simulink model "Task_No6_R2023a"  (R2023a)
settings: Solver=ode5  StartTime=0.0  StopTime=3600*24*7  FixedStep=1  RelTol=1e-3
InitFcn:
  | PARAMETERS;
StartFcn:
  | PARAMETERS;
values from neighbouring files (symbols this model uses):
  Conv_C_to_K = 273.15    [PARAMETERS.m]
  P_AC_AIR_FLOW = 1    [PARAMETERS.m]
  P_CP_AIR = 1012    [PARAMETERS.m]
  P_DENSITY_AIR = 1.2041    [PARAMETERS.m]
  P_DENSITY_BRICK = 2/(10^-3)    (= 2000)    [PARAMETERS.m]
  P_DENSITY_PUR = 150    [PARAMETERS.m]
  P_EM_GLASS = 0.94    [PARAMETERS.m]
  P_EM_WALL = 0.94    [PARAMETERS.m]
  P_HANDLER_AIR_FLOW = 0.1    [PARAMETERS.m]
  P_HUMAN = 100    [PARAMETERS.m]
  P_INIT_CO2 = 420    [PARAMETERS.m]
  P_M_HUMAN_CO2 = 0.02*P_DENSITY_CO2/3600    (= 1.1e-05)    [PARAMETERS.m]
  P_M_HUMAN_VAPOR = 500*10^-3/(24*3600)    (= 5.78703703704e-06)    [PARAMETERS.m]
  P_M_WINDOW_SPEC = 20    [PARAMETERS.m]
  P_THICK_BRICK = 0.175    [PARAMETERS.m]
  P_THICK_PUR = P_THICK_WALL - P_THICK_BRICK    (= 0.125)    [PARAMETERS.m]
  RH_INIT_BDR = 40    [PARAMETERS.m]
  T_BREATH = 34    [PARAMETERS.m]
  T_COOLER = 12    [PARAMETERS.m]
  T_HEATER = 50    [PARAMETERS.m]
  T_INIT_BDR = 22    [PARAMETERS.m]
  T_INIT_OUT = 2.9    [PARAMETERS.m]
  U_WALL = 0.32    [PARAMETERS.m]
  U_WINDOW = 3.0    (= 3)    [PARAMETERS.m]
undefined symbols (not defined in the file or in its folder): P_AREA_BATH, P_AREA_BDR1, P_AREA_BDR2, P_AREA_EAST_WALL_BATH, P_AREA_EAST_WALL_BDR2, P_AREA_EAST_WALL_KIT, P_AREA_HALL, P_AREA_KIT, P_AREA_LVR, P_AREA_NORTH_WALL_BATH, P_AREA_NORTH_WALL_BDR1, P_AREA_NORTH_WALL_BDR2, P_AREA_OUTER_WALL_BATH, P_AREA_OUTER_WALL_BDR1, P_AREA_OUTER_WALL_BDR2, P_AREA_OUTER_WALL_HALL, P_AREA_OUTER_WALL_KIT, P_AREA_OUTER_WALL_LVR, P_AREA_SOUTH_WALL_KIT, P_AREA_SOUTH_WALL_LVR, P_AREA_WALL_BATH_KIT, P_AREA_WALL_BDR1_BDR2, P_AREA_WALL_BDR1_HALL, P_AREA_WALL_BDR2_BATH, P_AREA_WALL_BDR2_HALL, P_AREA_WALL_HALL_BATH, P_AREA_WALL_HALL_LVR, P_AREA_WALL_LVR_KIT, P_AREA_WIN_BATH, P_AREA_WIN_BDRS, P_AREA_WIN_KIT, P_AREA_WIN_LVR, P_M_AIR_BATH, P_M_AIR_BDR1, P_M_AIR_BDR2, P_M_AIR_HALL, P_M_AIR_KIT, P_M_AIR_LVR, TBL_SOL_EAST_01, TBL_SOL_EAST_02, TBL_SOL_EAST_03, TBL_SOL_EAST_04, TBL_SOL_EAST_05, TBL_SOL_EAST_06, TBL_SOL_EAST_07, TBL_SOL_EAST_08, TBL_SOL_EAST_09, TBL_SOL_EAST_10, TBL_SOL_EAST_11, TBL_SOL_EAST_12, TBL_SOL_NORTH_01, TBL_SOL_NORTH_02, TBL_SOL_NORTH_03, TBL_SOL_NORTH_04, TBL_SOL_NORTH_05, TBL_SOL_NORTH_06, TBL_SOL_NORTH_07, TBL_SOL_NORTH_08, TBL_SOL_NORTH_09, TBL_SOL_NORTH_10 ... (+7)
libraries: fl_lib x166, nesl_utility x88, slpidlib x3
(part 3 of 5)

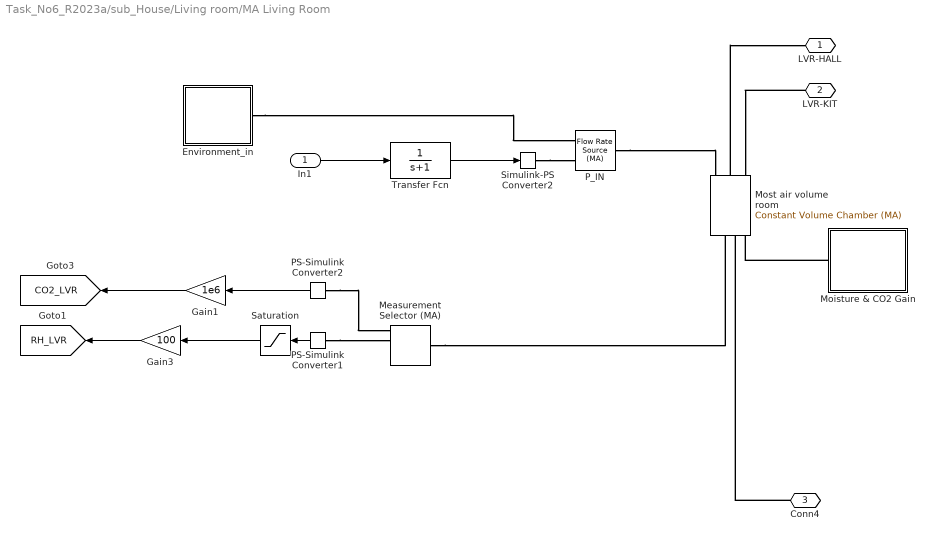
== system Task_No6_R2023a/sub_House/Living room/MA Living Room ==
  In1 : Inport
  Environment_in : Subsystem
  Gain1 : Gain  Gain=1e6
  Gain3 : Gain  Gain=100
  Measurement Selector (MA) : fl_lib/Moist Air/Sensors/Measurement Selector (MA)  moisture_spec=foundation.enum.moisture_spec.relative_humidity  trace_gas_spec=foundation.enum.trace_gas_spec.mass_fraction
  Moisture & CO2 Gain : Subsystem
  Most air volume room : fl_lib/Moist Air/Elements/Constant Volume Chamber (MA)  volume=P_M_AIR_LVR/P_DENSITY_AIR m^3  num_ports=foundation.enum.num_ports.three  area_A=P_AREA_DUCT m^2  area_B=P_AREA_DBL_DOOR m^2  area_C=P_AREA_DBL_DOOR m^2  area_D=0.01 m^2  RH_ws=1  time_constant=1 s  moisture_trace_gas_source=foundation.enum.moisture_trace_gas_source.controlled  moisture_source_spec=foundation.enum.moisture_source_spec.vapor  moisture_mass_flow=0 kg/s  moisture_temperature_spec=foundation.enum.temperature_spec.atmospheric  moisture_temperature=293.15 K  trace_gas_mass_flow=0 kg/s  trace_gas_temperature_spec=foundation.enum.temperature_spec.atmospheric  trace_gas_temperature=293.15 K  p_I_specify=on  p_I_priority=High  p_I=0.101325 MPa  p_I_nominal_specify=off  p_I_nominal_unit=MPa  p_I_nominal_value=1  T_I_specify=on  T_I_priority=High  T_I=T_INIT_BDR degC  T_I_nominal_specify=off  T_I_nominal_unit=K  T_I_nominal_value=1  RH_I_specify=on  RH_I_priority=High  RH_I=RH_INIT_BDR/100  RH_I_nominal_specify=off  RH_I_nominal_unit=1  RH_I_nominal_value=1  x_w_I_specify=off  x_w_I_priority=None  x_w_I=0  x_w_I_nominal_specify=off  x_w_I_nominal_unit=1  x_w_I_nominal_value=1  y_w_I_specify=off  y_w_I_priority=None  y_w_I=0  y_w_I_nominal_specify=off  y_w_I_nominal_unit=1  y_w_I_nominal_value=1  HR_I_specify=off  HR_I_priority=None  HR_I=0  HR_I_nominal_specify=off  HR_I_nominal_unit=1  HR_I_nominal_value=1  x_g_I_specify=on  x_g_I_priority=High  x_g_I=P_INIT_CO2/1e6  x_g_I_nominal_specify=off  x_g_I_nominal_unit=1  x_g_I_nominal_value=1  y_g_I_specify=off  y_g_I_priority=None  y_g_I=0  y_g_I_nominal_specify=off  y_g_I_nominal_unit=1  y_g_I_nominal_value=1
      settings: InternalSimscapePortConfiguration="{\"Bottom\":[],\"Left\":[{\"id\":\"A\",\"label\":\"A\",\"type\":\"foundation.moist_air.moist_air\"},{\"id\":\"B\",\"label\":\"B\",\"type\":\"foundation.moist_air.moist_air\"},{\"id\":\"C\",\"label\":\"C\",\"type\":\"foundation.moist_air.moist_air\"}],\"Right\":[{\"id\":\"W\",\"label\":\"W\",\"type\":\"output\"},{\"id\":\"F\",\"label\":\"F\",\"type\":\"output\"},{\"id\":\"H\",\"label\":\"H\",\"type\":\"foundation.thermal.thermal\"},{\"id\":\"S\",\"label\":\"S\",\"type\":\"foundation.moist_air.moist_air_source\"}],\"Top\":[]}"
  PS-Simulink Converter1 : nesl_utility/PS-Simulink Converter  PhysicalDomain=network_engine_domain  SubClassName=ps_output  LeftPortType=input  RightPortType=output  PseudoPeriodic=off  Frequencies=[]  VectorFormat=inherit  Unit=inherit  AffineConversion=off
  PS-Simulink Converter2 : nesl_utility/PS-Simulink Converter  PhysicalDomain=network_engine_domain  SubClassName=ps_output  LeftPortType=input  RightPortType=output  PseudoPeriodic=off  Frequencies=[]  VectorFormat=inherit  Unit=inherit  AffineConversion=off
  P_IN : fl_lib/Moist Air/Sources/Flow Rate Source (MA)  source_type=foundation.enum.constant_controlled.controlled  flow_type=foundation.enum.mass_volumetric_flow.mass  mass_flow=0 kg/s  volumetric_flow=0 m^3/s  volumetric_flow_conditions=foundation.enum.volumetric_flow_conditions.actual  p_std=0.101325 MPa  T_std=20 degC  RH_std=0.65  power_spec=foundation.enum.power_spec.isentropic  area_A=P_AREA_DUCT m^2  area_B=P_AREA_DUCT m^2
      settings: InternalSimscapePortConfiguration="{\"Bottom\":[],\"Left\":[{\"id\":\"A\",\"label\":\"A\",\"type\":\"foundation.moist_air.moist_air\"},{\"id\":\"M\",\"label\":\"M\",\"type\":\"input\"}],\"Right\":[{\"id\":\"B\",\"label\":\"B\",\"type\":\"foundation.moist_air.moist_air\"}],\"Top\":[]}"
  Saturation : Saturate  UpperLimit=1  LowerLimit=0
  Simulink-PS Converter2 : nesl_utility/Simulink-PS Converter  PhysicalDomain=network_engine_domain  SubClassName=ps_input  LeftPortType=input  RightPortType=output  PseudoPeriodic=off  Frequencies=[]  NoiseDistribution=none  NoiseParameters=[]  Unit=1  AffineConversion=off  FilteringAndDerivatives=provide  SimscapeFilterOrder=1  InputFilterTimeConstant=0.001  UdotUserProvided=0
  Transfer Fcn : TransferFcn  Denominator=[1 1]
  LVR-HALL : PMIOPort  Side=Left
  LVR-KIT : PMIOPort  Port=2  Side=Left
  Conn4 : PMIOPort  Port=3  Side=Right
  tag scope: CO2_LVR=global, RH_LVR=global
  wires:
  PS-Simulink Converter1/1 -> Saturation/1
  PS-Simulink Converter2/1 -> Gain1/1
  Saturation/1 -> Gain3/1
  Gain3/1 -> [RH_LVR]
  Gain1/1 -> [CO2_LVR]
  In1/1 -> Transfer Fcn/1
  Transfer Fcn/1 -> Simulink-PS Converter2/1
  connections:
  PS-Simulink Converter1/LConn1 -- Measurement Selector (MA)/RConn3
  PS-Simulink Converter2/LConn1 -- Measurement Selector (MA)/RConn4
  Conn4/RConn1 -- Most air volume room/RConn3
  Measurement Selector (MA)/LConn1 -- Most air volume room/RConn2
  P_IN/RConn1 -- Most air volume room/LConn1
  Most air volume room/LConn2 -- LVR-HALL/RConn1
  Moisture & CO2 Gain/LConn1 -- Most air volume room/RConn4
  Environment_in/LConn1 -- P_IN/LConn1
  Simulink-PS Converter2/RConn1 -- P_IN/LConn2
  LVR-KIT/RConn1 -- Most air volume room/LConn3

== system Task_No6_R2023a/sub_House/Bathroom/Bathroom/Ceiling & Floor (Bath<->Above & Below) ==
  Ceiling-InAir : fl_lib/Thermal/Thermal Elements/Thermal Resistance  resistance=1/(U_CEIL*P_AREA_BATH) K/W  T_specify=off  T_priority=None  T=0 K  T_nominal_specify=off  T_nominal_unit=K  T_nominal_value=1  Q_specify=off  Q_priority=None  Q=0 W  Q_nominal_specify=off  Q_nominal_unit=W  Q_nominal_value=1
  Floor-InAir : fl_lib/Thermal/Thermal Elements/Thermal Resistance  resistance=1/(U_CEIL*P_AREA_BATH) K/W  T_specify=off  T_priority=None  T=0 K  T_nominal_specify=off  T_nominal_unit=K  T_nominal_value=1  Q_specify=off  Q_priority=None  Q=0 W  Q_nominal_specify=off  Q_nominal_unit=W  Q_nominal_value=1
  Conn1 : PMIOPort  Side=Left
  Conn2 : PMIOPort  Port=2  Side=Right
  connections:
  Floor-InAir/RConn1 -- Ceiling-InAir/RConn1 -- Conn2/RConn1
  Floor-InAir/LConn1 -- Ceiling-InAir/LConn1 -- Conn1/RConn1

== system Task_No6_R2023a/sub_House/Bathroom/Bathroom/Inside Enivornment Temperature ==
  T_ENV : Inport
  Constant2 : Constant  Value=Conv_C_to_K
  Controlled Temperature Source : fl_lib/Thermal/Thermal Sources/Controlled Temperature Source
  Simulink-PS Converter1 : nesl_utility/Simulink-PS Converter  PhysicalDomain=network_engine_domain  SubClassName=ps_input  LeftPortType=input  RightPortType=output  PseudoPeriodic=off  Frequencies=[]  NoiseDistribution=none  NoiseParameters=[]  Unit=1  AffineConversion=off  FilteringAndDerivatives=provide  SimscapeFilterOrder=1  InputFilterTimeConstant=0.001  UdotUserProvided=0
  Sum : Sum  Inputs=|++
  Thermal Reference1 : fl_lib/Thermal/Thermal Elements/Thermal Reference
  Conn1 : PMIOPort  Side=Left
  wires:
  T_ENV/1 -> Sum/1
  Constant2/1 -> Sum/2
  Sum/1 -> Simulink-PS Converter1/1
  connections:
  Controlled Temperature Source/LConn1 -- Conn1/RConn1
  Simulink-PS Converter1/RConn1 -- Controlled Temperature Source/RConn1
  Thermal Reference1/LConn1 -- Controlled Temperature Source/RConn2

== system Task_No6_R2023a/sub_House/Bathroom/Bathroom/Outside Temperature ==
  T_OUT : Inport
  Constant2 : Constant  Value=Conv_C_to_K
  Controlled Temperature Source : fl_lib/Thermal/Thermal Sources/Controlled Temperature Source
  Simulink-PS Converter1 : nesl_utility/Simulink-PS Converter  PhysicalDomain=network_engine_domain  SubClassName=ps_input  LeftPortType=input  RightPortType=output  PseudoPeriodic=off  Frequencies=[]  NoiseDistribution=none  NoiseParameters=[]  Unit=1  AffineConversion=off  FilteringAndDerivatives=provide  SimscapeFilterOrder=1  InputFilterTimeConstant=0.001  UdotUserProvided=0
  Sum : Sum  Inputs=|++
  Thermal Reference1 : fl_lib/Thermal/Thermal Elements/Thermal Reference
  Conn1 : PMIOPort  Side=Left
  wires:
  Sum/1 -> Simulink-PS Converter1/1
  Constant2/1 -> Sum/2
  T_OUT/1 -> Sum/1
  connections:
  Thermal Reference1/LConn1 -- Controlled Temperature Source/RConn2
  Simulink-PS Converter1/RConn1 -- Controlled Temperature Source/RConn1
  Controlled Temperature Source/LConn1 -- Conn1/RConn1

== system Task_No6_R2023a/sub_House/Bathroom/Bathroom/SOLAR__WALL ==
  Add : Sum
  Constant : Constant  Value=P_AREA_NORTH_WALL_BATH
  Constant1 : Constant  Value=P_EM_WALL
  Constant2 : Constant  Value=P_AREA_EAST_WALL_BATH
  Constant3 : Constant  Value=P_EM_WALL
  Controlled Heat Flow Rate Source : fl_lib/Thermal/Thermal Sources/Controlled Heat Flow Rate Source
  Product : Product  Inputs=3
  Product1 : Product  Inputs=3
  Simulink-PS Converter : nesl_utility/Simulink-PS Converter  PhysicalDomain=network_engine_domain  SubClassName=ps_input  LeftPortType=input  RightPortType=output  PseudoPeriodic=off  Frequencies=[]  NoiseDistribution=none  NoiseParameters=[]  Unit=1  AffineConversion=off  FilteringAndDerivatives=provide  SimscapeFilterOrder=1  InputFilterTimeConstant=0.001  UdotUserProvided=0
  Thermal Reference : fl_lib/Thermal/Thermal Elements/Thermal Reference
  Conn1 : PMIOPort  Side=Left
  wires:
  Constant/1 -> Product/2
  Constant1/1 -> Product/1
  [SOL_NORTH] -> Product/3
  Product/1 -> Add/1
  Constant3/1 -> Product1/1
  [SOL_EAST] -> Product1/3
  Constant2/1 -> Product1/2
  Add/1 -> Simulink-PS Converter/1
  Product1/1 -> Add/2
  connections:
  Controlled Heat Flow Rate Source/LConn1 -- Conn1/RConn1
  Simulink-PS Converter/RConn1 -- Controlled Heat Flow Rate Source/RConn1
  Thermal Reference/LConn1 -- Controlled Heat Flow Rate Source/RConn2

== system Task_No6_R2023a/sub_House/Bathroom/Bathroom/SOLAR__WINDOW ==
  Constant : Constant  Value=P_AREA_WIN_BATH
  Constant1 : Constant  Value=P_EM_GLASS
  Controlled Heat Flow Rate Source : fl_lib/Thermal/Thermal Sources/Controlled Heat Flow Rate Source
  Product : Product  Inputs=3
  Simulink-PS Converter : nesl_utility/Simulink-PS Converter  PhysicalDomain=network_engine_domain  SubClassName=ps_input  LeftPortType=input  RightPortType=output  PseudoPeriodic=off  Frequencies=[]  NoiseDistribution=none  NoiseParameters=[]  Unit=1  AffineConversion=off  FilteringAndDerivatives=provide  SimscapeFilterOrder=1  InputFilterTimeConstant=0.001  UdotUserProvided=0
  Thermal Reference : fl_lib/Thermal/Thermal Elements/Thermal Reference
  Conn1 : PMIOPort  Side=Left
  wires:
  Product/1 -> Simulink-PS Converter/1
  [SOL_EAST] -> Product/3
  Constant1/1 -> Product/1
  Constant/1 -> Product/2
  connections:
  Thermal Reference/LConn1 -- Controlled Heat Flow Rate Source/RConn2
  Simulink-PS Converter/RConn1 -- Controlled Heat Flow Rate Source/RConn1
  Controlled Heat Flow Rate Source/LConn1 -- Conn1/RConn1

== system Task_No6_R2023a/sub_House/Bathroom/Bathroom/TEMP_01 ==
  Constant2 : Constant  Value=Conv_C_to_K
  PS-Simulink Converter : nesl_utility/PS-Simulink Converter  PhysicalDomain=network_engine_domain  SubClassName=ps_output  LeftPortType=input  RightPortType=output  PseudoPeriodic=off  Frequencies=[]  VectorFormat=inherit  Unit=inherit  AffineConversion=off
  Sum : Sum  Inputs=|+-
  Temperature Sensor : fl_lib/Thermal/Thermal Sensors/Temperature Sensor  temperature_measure=foundation.enum.MeasurementReference.difference
  Thermal Reference2 : fl_lib/Thermal/Thermal Elements/Thermal Reference
  PS : PMIOPort  Side=Left
  Sim : Outport
  wires:
  Sum/1 -> Sim/1
  PS-Simulink Converter/1 -> Sum/1
  Constant2/1 -> Sum/2
  connections:
  Thermal Reference2/LConn1 -- Temperature Sensor/RConn1
  PS-Simulink Converter/LConn1 -- Temperature Sensor/RConn2
  PS/RConn1 -- Temperature Sensor/LConn1

== system Task_No6_R2023a/sub_House/Bathroom/Bathroom/Wall (Bath<->Outside) ==
  InAir-Wall : fl_lib/Thermal/Thermal Elements/Thermal Resistance  resistance=1/(U_WALL*P_AREA_OUTER_WALL_BATH)/2 K/W  T_specify=off  T_priority=None  T=0 K  T_nominal_specify=off  T_nominal_unit=K  T_nominal_value=1  Q_specify=off  Q_priority=None  Q=0 W  Q_nominal_specify=off  Q_nominal_unit=W  Q_nominal_value=1
  Thermal Mass of wall : fl_lib/Thermal/Thermal Elements/Thermal Mass  mass_type=foundation.enum.constant_variable.constant  mass=P_AREA_OUTER_WALL_BATH*(P_THICK_BRICK*P_DENSITY_BRICK+P_THICK_PUR*P_DENSITY_PUR) kg  sp_heat=P_CP_WALL J/(K*kg)  mass_min=1e-6 kg  num_ports=foundation.enum.numPorts2.one  m_specify=off  m_priority=High  m=1 kg  m_nominal_specify=off  m_nominal_unit=kg  m_nominal_value=1  T_specify=on  T_priority=High  T=T_INIT_BDR degC  T_nominal_specify=off  T_nominal_unit=K  T_nominal_value=1  Q_specify=off  Q_priority=None  Q=0 W  Q_nominal_specify=off  Q_nominal_unit=W  Q_nominal_value=1
  Wall-OutAir : fl_lib/Thermal/Thermal Elements/Thermal Resistance  resistance=1/(U_WALL*P_AREA_OUTER_WALL_BATH)/2 K/W  T_specify=off  T_priority=None  T=0 K  T_nominal_specify=off  T_nominal_unit=K  T_nominal_value=1  Q_specify=off  Q_priority=None  Q=0 W  Q_nominal_specify=off  Q_nominal_unit=W  Q_nominal_value=1
  Conn1 : PMIOPort  Side=Left
  Conn3 : PMIOPort  Port=2  Side=Right
  Conn2 : PMIOPort  Port=3  Side=Right
  connections:
  Conn1/RConn1 -- InAir-Wall/LConn1
  InAir-Wall/RConn1 -- Conn3/RConn1 -- Thermal Mass of wall/LConn1 -- Wall-OutAir/LConn1
  Wall-OutAir/RConn1 -- Conn2/RConn1

== system Task_No6_R2023a/sub_House/Bathroom/Bathroom/Window (Bath<->Outside) ==
  InAir-Window : fl_lib/Thermal/Thermal Elements/Thermal Resistance  resistance=1/(U_WINDOW*P_AREA_WIN_BATH)/2 K/W  T_specify=off  T_priority=None  T=0 K  T_nominal_specify=off  T_nominal_unit=K  T_nominal_value=1  Q_specify=off  Q_priority=None  Q=0 W  Q_nominal_specify=off  Q_nominal_unit=W  Q_nominal_value=1
  Thermal Mass of window : fl_lib/Thermal/Thermal Elements/Thermal Mass  mass_type=foundation.enum.constant_variable.constant  mass=P_M_WINDOW_SPEC*P_AREA_WIN_BATH kg  sp_heat=P_CP_GLASS J/(K*kg)  mass_min=1e-6 kg  num_ports=foundation.enum.numPorts2.one  m_specify=off  m_priority=High  m=1 kg  m_nominal_specify=off  m_nominal_unit=kg  m_nominal_value=1  T_specify=on  T_priority=High  T=T_INIT_BDR degC  T_nominal_specify=off  T_nominal_unit=K  T_nominal_value=1  Q_specify=off  Q_priority=None  Q=0 W  Q_nominal_specify=off  Q_nominal_unit=W  Q_nominal_value=1
  Window-OutAir : fl_lib/Thermal/Thermal Elements/Thermal Resistance  resistance=1/(U_WINDOW*P_AREA_WIN_BATH)/2 K/W  T_specify=off  T_priority=None  T=0 K  T_nominal_specify=off  T_nominal_unit=K  T_nominal_value=1  Q_specify=off  Q_priority=None  Q=0 W  Q_nominal_specify=off  Q_nominal_unit=W  Q_nominal_value=1
  Conn1 : PMIOPort  Side=Right
  Conn2 : PMIOPort  Port=2  Side=Left
  Conn3 : PMIOPort  Port=3  Side=Right
  connections:
  Thermal Mass of window/LConn1 -- Conn3/RConn1 -- Window-OutAir/LConn1 -- InAir-Window/RConn1
  Conn1/RConn1 -- Window-OutAir/RConn1
  Conn2/RConn1 -- InAir-Window/LConn1

== system Task_No6_R2023a/sub_House/Bathroom/MA Bathroom/Environment_out ==
  Constant1 : Constant  Value=P_INIT_CO2
  Constant4 : Constant  Value=1e5
  Constant6 : Constant  Value=Conv_C_to_K
  Controlled Reservoir (MA) : fl_lib/Moist Air/Elements/Controlled Reservoir (MA)  moisture_spec=foundation.enum.moistureSpec.RelativeHumidity  trace_gas_spec=foundation.enum.trace_gas_spec.mass_fraction  RH_ws=1  area_A=P_AREA_DUCT m^2  input_error_spec=foundation.enum.input_range_error.warn
      settings: InternalSimscapePortConfiguration="{\"Bottom\":[],\"Left\":[{\"id\":\"A\",\"label\":\"A\",\"type\":\"foundation.moist_air.moist_air\"}],\"Right\":[{\"id\":\"T\",\"label\":\"T\",\"type\":\"input\"},{\"id\":\"P\",\"label\":\"P\",\"type\":\"input\"},{\"id\":\"W\",\"label\":\"W\",\"type\":\"input\"},{\"id\":\"G\",\"label\":\"G\",\"type\":\"input\"}],\"Top\":[]}"
  Gain : Gain  Gain=1/100
  Gain2 : Gain  Gain=1e-6
  Simulink-PS Converter{3,5..7} (4 alike) : nesl_utility/Simulink-PS Converter  PhysicalDomain=network_engine_domain  SubClassName=ps_input  LeftPortType=input  RightPortType=output  PseudoPeriodic=off  Frequencies=[]  NoiseDistribution=none  NoiseParameters=[]  Unit=1  AffineConversion=off  FilteringAndDerivatives=provide  SimscapeFilterOrder=1  InputFilterTimeConstant=0.001  UdotUserProvided=0
  Sum2 : Sum  Inputs=|++
  Conn1 : PMIOPort  Side=Left
  wires:
  Constant1/1 -> Gain2/1
  Constant6/1 -> Sum2/2
  Gain/1 -> Simulink-PS Converter6/1
  Constant4/1 -> Simulink-PS Converter5/1
  Gain2/1 -> Simulink-PS Converter7/1
  Sum2/1 -> Simulink-PS Converter3/1
  [T_OUT] -> Sum2/1
  [RH_OUT] -> Gain/1
  connections:
  Simulink-PS Converter3/RConn1 -- Controlled Reservoir (MA)/RConn1
  Simulink-PS Converter7/RConn1 -- Controlled Reservoir (MA)/RConn4
  Controlled Reservoir (MA)/LConn1 -- Conn1/RConn1
  Simulink-PS Converter5/RConn1 -- Controlled Reservoir (MA)/RConn2
  Simulink-PS Converter6/RConn1 -- Controlled Reservoir (MA)/RConn3

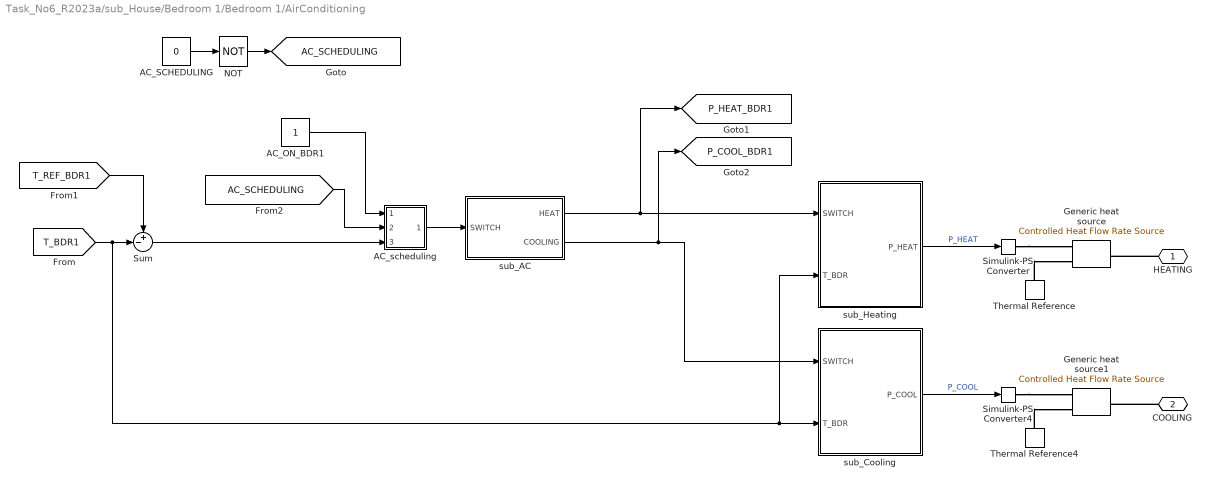
== system Task_No6_R2023a/sub_House/Bedroom 1/Bedroom 1/AirConditioning ==
  AC_ON_BDR1 : Constant
  AC_SCHEDULING : Constant  Value=0
  AC_scheduling : Subsystem
  Generic heat source : fl_lib/Thermal/Thermal Sources/Controlled Heat Flow Rate Source
  Generic heat source1 : fl_lib/Thermal/Thermal Sources/Controlled Heat Flow Rate Source
  NOT : Logic  Operator=NOT  IconShape=distinctive  AllPortsSameDT=off  OutDataTypeStr=boolean
  Simulink-PS Converter : nesl_utility/Simulink-PS Converter  PhysicalDomain=network_engine_domain  SubClassName=ps_input  LeftPortType=input  RightPortType=output  PseudoPeriodic=off  Frequencies=[]  NoiseDistribution=none  NoiseParameters=[]  Unit=1  AffineConversion=off  FilteringAndDerivatives=provide  SimscapeFilterOrder=1  InputFilterTimeConstant=0.001  UdotUserProvided=0
  Simulink-PS Converter4 : nesl_utility/Simulink-PS Converter  PhysicalDomain=network_engine_domain  SubClassName=ps_input  LeftPortType=input  RightPortType=output  PseudoPeriodic=off  Frequencies=[]  NoiseDistribution=none  NoiseParameters=[]  Unit=1  AffineConversion=off  FilteringAndDerivatives=provide  SimscapeFilterOrder=1  InputFilterTimeConstant=0.001  UdotUserProvided=0
  Sum : Sum  Inputs=+-|
  Thermal Reference : fl_lib/Thermal/Thermal Elements/Thermal Reference
  Thermal Reference4 : fl_lib/Thermal/Thermal Elements/Thermal Reference
  sub_AC : Subsystem
  sub_Cooling : Subsystem
  sub_Heating : Subsystem
  HEATING : PMIOPort  Side=Right
  COOLING : PMIOPort  Port=2  Side=Right
  tag scope: AC_SCHEDULING=global, P_COOL_BDR1=global, P_HEAT_BDR1=global
  wires:
  sub_AC/2(COOLING) -> [P_COOL_BDR1], sub_Cooling/1(SWITCH)
  sub_AC/1(HEAT) -> [P_HEAT_BDR1], sub_Heating/1(SWITCH)
  [T_BDR1] -> sub_Heating/2(T_BDR), sub_Cooling/2(T_BDR), Sum/2
  sub_Heating/1(P_HEAT) -> Simulink-PS Converter/1  "P_HEAT"
  sub_Cooling/1(P_COOL) -> Simulink-PS Converter4/1  "P_COOL"
  [T_REF_BDR1] -> Sum/1
  AC_ON_BDR1/1 -> AC_scheduling/1(In1)
  Sum/1 -> AC_scheduling/3(In2)
  AC_scheduling/1(Out1) -> sub_AC/1(SWITCH)
  AC_SCHEDULING/1 -> NOT/1
  [AC_SCHEDULING] -> AC_scheduling/2(In3)
  NOT/1 -> [AC_SCHEDULING]
  connections:
  Thermal Reference4/LConn1 -- Generic heat source1/RConn2
  Thermal Reference/LConn1 -- Generic heat source/RConn2
  Simulink-PS Converter4/RConn1 -- Generic heat source1/RConn1
  Simulink-PS Converter/RConn1 -- Generic heat source/RConn1
  HEATING/RConn1 -- Generic heat source/LConn1
  COOLING/RConn1 -- Generic heat source1/LConn1

== system Task_No6_R2023a/sub_House/Bedroom 1/Bedroom 1/Ceiling & Floor (BDR1<->Above & Below) ==
  Ceiling-InAir : fl_lib/Thermal/Thermal Elements/Thermal Resistance  resistance=1/(U_CEIL*P_AREA_BDR1) K/W  T_specify=off  T_priority=None  T=0 K  T_nominal_specify=off  T_nominal_unit=K  T_nominal_value=1  Q_specify=off  Q_priority=None  Q=0 W  Q_nominal_specify=off  Q_nominal_unit=W  Q_nominal_value=1
  Floor-InAir : fl_lib/Thermal/Thermal Elements/Thermal Resistance  resistance=1/(U_CEIL*P_AREA_BDR1) K/W  T_specify=off  T_priority=None  T=0 K  T_nominal_specify=off  T_nominal_unit=K  T_nominal_value=1  Q_specify=off  Q_priority=None  Q=0 W  Q_nominal_specify=off  Q_nominal_unit=W  Q_nominal_value=1
  Conn1 : PMIOPort  Side=Left
  Conn2 : PMIOPort  Port=2  Side=Right
  connections:
  Ceiling-InAir/RConn1 -- Conn2/RConn1 -- Floor-InAir/RConn1
  Ceiling-InAir/LConn1 -- Conn1/RConn1 -- Floor-InAir/LConn1

== system Task_No6_R2023a/sub_House/Bedroom 1/Bedroom 1/Heat source human ==
  Constant : Constant  Value=P_HUMAN
  Controlled Heat Flow Rate Source : fl_lib/Thermal/Thermal Sources/Controlled Heat Flow Rate Source
  Product : Product
  Simulink-PS Converter : nesl_utility/Simulink-PS Converter  PhysicalDomain=network_engine_domain  SubClassName=ps_input  LeftPortType=input  RightPortType=output  PseudoPeriodic=off  Frequencies=[]  NoiseDistribution=none  NoiseParameters=[]  Unit=1  AffineConversion=off  FilteringAndDerivatives=provide  SimscapeFilterOrder=1  InputFilterTimeConstant=0.001  UdotUserProvided=0
  Thermal Reference : fl_lib/Thermal/Thermal Elements/Thermal Reference
  Conn1 : PMIOPort  Side=Left
  wires:
  [N_BDR1] -> Product/1
  Constant/1 -> Product/2
  Product/1 -> Simulink-PS Converter/1
  connections:
  Thermal Reference/LConn1 -- Controlled Heat Flow Rate Source/RConn2
  Simulink-PS Converter/RConn1 -- Controlled Heat Flow Rate Source/RConn1
  Controlled Heat Flow Rate Source/LConn1 -- Conn1/RConn1

== system Task_No6_R2023a/sub_House/Bedroom 1/Bedroom 1/Inside Enivornment Temperature ==
  T_ENV : Inport
  Constant2 : Constant  Value=Conv_C_to_K
  Controlled Temperature Source : fl_lib/Thermal/Thermal Sources/Controlled Temperature Source
  Simulink-PS Converter1 : nesl_utility/Simulink-PS Converter  PhysicalDomain=network_engine_domain  SubClassName=ps_input  LeftPortType=input  RightPortType=output  PseudoPeriodic=off  Frequencies=[]  NoiseDistribution=none  NoiseParameters=[]  Unit=1  AffineConversion=off  FilteringAndDerivatives=provide  SimscapeFilterOrder=1  InputFilterTimeConstant=0.001  UdotUserProvided=0
  Sum : Sum  Inputs=|++
  Thermal Reference1 : fl_lib/Thermal/Thermal Elements/Thermal Reference
  Conn1 : PMIOPort  Side=Left
  wires:
  T_ENV/1 -> Sum/1
  Constant2/1 -> Sum/2
  Sum/1 -> Simulink-PS Converter1/1
  connections:
  Controlled Temperature Source/LConn1 -- Conn1/RConn1
  Simulink-PS Converter1/RConn1 -- Controlled Temperature Source/RConn1
  Thermal Reference1/LConn1 -- Controlled Temperature Source/RConn2

== system Task_No6_R2023a/sub_House/Bedroom 1/Bedroom 1/Outside Temperature ==
  T_OUT : Inport
  Constant2 : Constant  Value=Conv_C_to_K
  Controlled Temperature Source : fl_lib/Thermal/Thermal Sources/Controlled Temperature Source
  Simulink-PS Converter1 : nesl_utility/Simulink-PS Converter  PhysicalDomain=network_engine_domain  SubClassName=ps_input  LeftPortType=input  RightPortType=output  PseudoPeriodic=off  Frequencies=[]  NoiseDistribution=none  NoiseParameters=[]  Unit=1  AffineConversion=off  FilteringAndDerivatives=provide  SimscapeFilterOrder=1  InputFilterTimeConstant=0.001  UdotUserProvided=0
  Sum : Sum  Inputs=|++
  Thermal Reference1 : fl_lib/Thermal/Thermal Elements/Thermal Reference
  Conn1 : PMIOPort  Side=Left
  wires:
  Sum/1 -> Simulink-PS Converter1/1
  Constant2/1 -> Sum/2
  T_OUT/1 -> Sum/1
  connections:
  Thermal Reference1/LConn1 -- Controlled Temperature Source/RConn2
  Simulink-PS Converter1/RConn1 -- Controlled Temperature Source/RConn1
  Controlled Temperature Source/LConn1 -- Conn1/RConn1

== system Task_No6_R2023a/sub_House/Bedroom 1/Bedroom 1/SOLAR__WALL ==
  Constant : Constant  Value=P_AREA_NORTH_WALL_BDR1
  Constant1 : Constant  Value=P_EM_WALL
  Controlled Heat Flow Rate Source : fl_lib/Thermal/Thermal Sources/Controlled Heat Flow Rate Source
  Product : Product  Inputs=3
  Simulink-PS Converter : nesl_utility/Simulink-PS Converter  PhysicalDomain=network_engine_domain  SubClassName=ps_input  LeftPortType=input  RightPortType=output  PseudoPeriodic=off  Frequencies=[]  NoiseDistribution=none  NoiseParameters=[]  Unit=1  AffineConversion=off  FilteringAndDerivatives=provide  SimscapeFilterOrder=1  InputFilterTimeConstant=0.001  UdotUserProvided=0
  Thermal Reference : fl_lib/Thermal/Thermal Elements/Thermal Reference
  Conn1 : PMIOPort  Side=Left
  wires:
  Constant/1 -> Product/2
  Constant1/1 -> Product/1
  [SOL_NORTH] -> Product/3
  Product/1 -> Simulink-PS Converter/1
  connections:
  Controlled Heat Flow Rate Source/LConn1 -- Conn1/RConn1
  Simulink-PS Converter/RConn1 -- Controlled Heat Flow Rate Source/RConn1
  Thermal Reference/LConn1 -- Controlled Heat Flow Rate Source/RConn2

== system Task_No6_R2023a/sub_House/Bedroom 1/Bedroom 1/SOLAR__WINDOW ==
  Constant : Constant  Value=P_AREA_WIN_BDRS
  Constant1 : Constant  Value=P_EM_GLASS
  Controlled Heat Flow Rate Source : fl_lib/Thermal/Thermal Sources/Controlled Heat Flow Rate Source
  Product : Product  Inputs=3
  Simulink-PS Converter : nesl_utility/Simulink-PS Converter  PhysicalDomain=network_engine_domain  SubClassName=ps_input  LeftPortType=input  RightPortType=output  PseudoPeriodic=off  Frequencies=[]  NoiseDistribution=none  NoiseParameters=[]  Unit=1  AffineConversion=off  FilteringAndDerivatives=provide  SimscapeFilterOrder=1  InputFilterTimeConstant=0.001  UdotUserProvided=0
  Thermal Reference : fl_lib/Thermal/Thermal Elements/Thermal Reference
  Conn1 : PMIOPort  Side=Left
  wires:
  Product/1 -> Simulink-PS Converter/1
  [SOL_NORTH] -> Product/3
  Constant1/1 -> Product/1
  Constant/1 -> Product/2
  connections:
  Thermal Reference/LConn1 -- Controlled Heat Flow Rate Source/RConn2
  Simulink-PS Converter/RConn1 -- Controlled Heat Flow Rate Source/RConn1
  Controlled Heat Flow Rate Source/LConn1 -- Conn1/RConn1

== system Task_No6_R2023a/sub_House/Bedroom 1/Bedroom 1/TEMP_01 ==
  Constant2 : Constant  Value=Conv_C_to_K
  PS-Simulink Converter : nesl_utility/PS-Simulink Converter  PhysicalDomain=network_engine_domain  SubClassName=ps_output  LeftPortType=input  RightPortType=output  PseudoPeriodic=off  Frequencies=[]  VectorFormat=inherit  Unit=inherit  AffineConversion=off
  Sum : Sum  Inputs=|+-
  Temperature Sensor : fl_lib/Thermal/Thermal Sensors/Temperature Sensor  temperature_measure=foundation.enum.MeasurementReference.difference
  Thermal Reference2 : fl_lib/Thermal/Thermal Elements/Thermal Reference
  PS : PMIOPort  Side=Left
  Sim : Outport
  wires:
  Sum/1 -> Sim/1
  PS-Simulink Converter/1 -> Sum/1
  Constant2/1 -> Sum/2
  connections:
  Thermal Reference2/LConn1 -- Temperature Sensor/RConn1
  PS-Simulink Converter/LConn1 -- Temperature Sensor/RConn2
  PS/RConn1 -- Temperature Sensor/LConn1

== system Task_No6_R2023a/sub_House/Bedroom 1/Bedroom 1/Wall (BDR1<->Outside) ==
  InAir-Wall : fl_lib/Thermal/Thermal Elements/Thermal Resistance  resistance=1/(U_WALL*P_AREA_OUTER_WALL_BDR1)/2 K/W  T_specify=off  T_priority=None  T=0 K  T_nominal_specify=off  T_nominal_unit=K  T_nominal_value=1  Q_specify=off  Q_priority=None  Q=0 W  Q_nominal_specify=off  Q_nominal_unit=W  Q_nominal_value=1
  Thermal Mass of wall : fl_lib/Thermal/Thermal Elements/Thermal Mass  mass_type=foundation.enum.constant_variable.constant  mass=P_AREA_OUTER_WALL_BDR1*(P_THICK_BRICK*P_DENSITY_BRICK+P_THICK_PUR*P_DENSITY_PUR) kg  sp_heat=P_CP_WALL J/(K*kg)  mass_min=1e-6 kg  num_ports=foundation.enum.numPorts2.one  m_specify=off  m_priority=High  m=1 kg  m_nominal_specify=off  m_nominal_unit=kg  m_nominal_value=1  T_specify=on  T_priority=High  T=T_INIT_BDR degC  T_nominal_specify=off  T_nominal_unit=K  T_nominal_value=1  Q_specify=off  Q_priority=None  Q=0 W  Q_nominal_specify=off  Q_nominal_unit=W  Q_nominal_value=1
  Wall-OutAir : fl_lib/Thermal/Thermal Elements/Thermal Resistance  resistance=1/(U_WALL*P_AREA_OUTER_WALL_BDR1)/2 K/W  T_specify=off  T_priority=None  T=0 K  T_nominal_specify=off  T_nominal_unit=K  T_nominal_value=1  Q_specify=off  Q_priority=None  Q=0 W  Q_nominal_specify=off  Q_nominal_unit=W  Q_nominal_value=1
  Conn1 : PMIOPort  Side=Left
  Conn3 : PMIOPort  Port=2  Side=Right
  Conn2 : PMIOPort  Port=3  Side=Right
  connections:
  Conn1/RConn1 -- InAir-Wall/LConn1
  InAir-Wall/RConn1 -- Conn3/RConn1 -- Thermal Mass of wall/LConn1 -- Wall-OutAir/LConn1
  Wall-OutAir/RConn1 -- Conn2/RConn1

== system Task_No6_R2023a/sub_House/Bedroom 1/Bedroom 1/Window (BDR1<->Outside) ==
  InAir-Window : fl_lib/Thermal/Thermal Elements/Thermal Resistance  resistance=1/(U_WINDOW*P_AREA_WIN_BDRS)/2 K/W  T_specify=off  T_priority=None  T=0 K  T_nominal_specify=off  T_nominal_unit=K  T_nominal_value=1  Q_specify=off  Q_priority=None  Q=0 W  Q_nominal_specify=off  Q_nominal_unit=W  Q_nominal_value=1
  Thermal Mass of window : fl_lib/Thermal/Thermal Elements/Thermal Mass  mass_type=foundation.enum.constant_variable.constant  mass=P_M_WINDOW_SPEC*P_AREA_WIN_BDRS kg  sp_heat=P_CP_GLASS J/(K*kg)  mass_min=1e-6 kg  num_ports=foundation.enum.numPorts2.one  m_specify=off  m_priority=High  m=1 kg  m_nominal_specify=off  m_nominal_unit=kg  m_nominal_value=1  T_specify=on  T_priority=High  T=T_INIT_BDR degC  T_nominal_specify=off  T_nominal_unit=K  T_nominal_value=1  Q_specify=off  Q_priority=None  Q=0 W  Q_nominal_specify=off  Q_nominal_unit=W  Q_nominal_value=1
  Window-OutAir : fl_lib/Thermal/Thermal Elements/Thermal Resistance  resistance=1/(U_WINDOW*P_AREA_WIN_BDRS)/2 K/W  T_specify=off  T_priority=None  T=0 K  T_nominal_specify=off  T_nominal_unit=K  T_nominal_value=1  Q_specify=off  Q_priority=None  Q=0 W  Q_nominal_specify=off  Q_nominal_unit=W  Q_nominal_value=1
  Conn1 : PMIOPort  Side=Right
  Conn2 : PMIOPort  Port=2  Side=Left
  Conn3 : PMIOPort  Port=3  Side=Right
  connections:
  Window-OutAir/LConn1 -- Thermal Mass of window/LConn1 -- Conn3/RConn1 -- InAir-Window/RConn1
  Conn1/RConn1 -- Window-OutAir/RConn1
  Conn2/RConn1 -- InAir-Window/LConn1

== system Task_No6_R2023a/sub_House/Bedroom 1/MA Bedroom 1/Environment_in ==
  Constant1 : Constant  Value=P_INIT_CO2
  Constant4 : Constant  Value=1e5
  Constant6 : Constant  Value=Conv_C_to_K
  Controlled Reservoir (MA) : fl_lib/Moist Air/Elements/Controlled Reservoir (MA)  moisture_spec=foundation.enum.moistureSpec.RelativeHumidity  trace_gas_spec=foundation.enum.trace_gas_spec.mass_fraction  RH_ws=1  area_A=P_AREA_DUCT m^2  input_error_spec=foundation.enum.input_range_error.warn
      settings: InternalSimscapePortConfiguration="{\"Bottom\":[],\"Left\":[{\"id\":\"A\",\"label\":\"A\",\"type\":\"foundation.moist_air.moist_air\"}],\"Right\":[{\"id\":\"T\",\"label\":\"T\",\"type\":\"input\"},{\"id\":\"P\",\"label\":\"P\",\"type\":\"input\"},{\"id\":\"W\",\"label\":\"W\",\"type\":\"input\"},{\"id\":\"G\",\"label\":\"G\",\"type\":\"input\"}],\"Top\":[]}"
  Gain : Gain  Gain=1/100
  Gain2 : Gain  Gain=1e-6
  Simulink-PS Converter{3,5..7} (4 alike) : nesl_utility/Simulink-PS Converter  PhysicalDomain=network_engine_domain  SubClassName=ps_input  LeftPortType=input  RightPortType=output  PseudoPeriodic=off  Frequencies=[]  NoiseDistribution=none  NoiseParameters=[]  Unit=1  AffineConversion=off  FilteringAndDerivatives=provide  SimscapeFilterOrder=1  InputFilterTimeConstant=0.001  UdotUserProvided=0
  Sum2 : Sum  Inputs=|++
  Conn1 : PMIOPort  Side=Left
  wires:
  [RH_OUT] -> Gain/1
  [T_OUT] -> Sum2/1
  Sum2/1 -> Simulink-PS Converter3/1
  Gain2/1 -> Simulink-PS Converter7/1
  Constant4/1 -> Simulink-PS Converter5/1
  Gain/1 -> Simulink-PS Converter6/1
  Constant6/1 -> Sum2/2
  Constant1/1 -> Gain2/1
  connections:
  Simulink-PS Converter6/RConn1 -- Controlled Reservoir (MA)/RConn3
  Simulink-PS Converter5/RConn1 -- Controlled Reservoir (MA)/RConn2
  Controlled Reservoir (MA)/LConn1 -- Conn1/RConn1
  Simulink-PS Converter7/RConn1 -- Controlled Reservoir (MA)/RConn4
  Simulink-PS Converter3/RConn1 -- Controlled Reservoir (MA)/RConn1

== system Task_No6_R2023a/sub_House/Bedroom 1/MA Bedroom 1/Moisture & CO2 Gain ==
  Constant : Constant  Value=T_BREATH
  Constant1 : Constant  Value=P_M_HUMAN_VAPOR
  Constant2 : Constant  Value=P_M_HUMAN_CO2
  Constant3 : Constant  Value=Conv_C_to_K
  Inhabitant CO2 Gain : fl_lib/Moist Air/Sources/Moisture & Trace Gas Sources/Trace Gas Source (MA)  source_type=foundation.enum.constant_controlled.controlled  trace_gas_mass_flow=P_M_HUMAN_CO2 kg/s  temperature_spec=foundation.enum.temperature_spec.specified  trace_gas_temperature=T_BREATH degC  Phi_S_specify=off  Phi_S_priority=None  Phi_S=0 kW  Phi_S_nominal_specify=off  Phi_S_nominal_unit=kW  Phi_S_nominal_value=1  mdot_g_S_specify=off  mdot_g_S_priority=None  mdot_g_S=0 kg/s  mdot_g_S_nominal_specify=off  mdot_g_S_nominal_unit=kg/s  mdot_g_S_nominal_value=1
      settings: InternalSimscapePortConfiguration="{\"Bottom\":[],\"Left\":[{\"id\":\"S\",\"label\":\"S\",\"type\":\"foundation.moist_air.moist_air_source\"}],\"Right\":[{\"id\":\"M\",\"label\":\"M\",\"type\":\"input\"},{\"id\":\"T\",\"label\":\"T\",\"type\":\"input\"}],\"Top\":[]}"
  Inhabitant Moisture Gain : fl_lib/Moist Air/Sources/Moisture & Trace Gas Sources/Moisture Source (MA)  source_type=foundation.enum.constant_controlled.controlled  moisture_source_spec=foundation.enum.moisture_source_spec.vapor  moisture_mass_flow=P_M_HUMAN_VAPOR kg/s  temperature_spec=foundation.enum.temperature_spec.specified  moisture_temperature=T_BREATH degC  Phi_S_specify=off  Phi_S_priority=None  Phi_S=0 kW  Phi_S_nominal_specify=off  Phi_S_nominal_unit=kW  Phi_S_nominal_value=1  mdot_w_S_specify=off  mdot_w_S_priority=None  mdot_w_S=0 kg/s  mdot_w_S_nominal_specify=off  mdot_w_S_nominal_unit=kg/s  mdot_w_S_nominal_value=1
      settings: InternalSimscapePortConfiguration="{\"Bottom\":[],\"Left\":[{\"id\":\"S\",\"label\":\"S\",\"type\":\"foundation.moist_air.moist_air_source\"}],\"Right\":[{\"id\":\"M\",\"label\":\"M\",\"type\":\"input\"},{\"id\":\"T\",\"label\":\"T\",\"type\":\"input\"}],\"Top\":[]}"
  Product : Product
  Product1 : Product
  Simulink-PS Converter : nesl_utility/Simulink-PS Converter  PhysicalDomain=network_engine_domain  SubClassName=ps_input  LeftPortType=input  RightPortType=output  PseudoPeriodic=off  Frequencies=[]  NoiseDistribution=none  NoiseParameters=[]  Unit=1  AffineConversion=off  FilteringAndDerivatives=provide  SimscapeFilterOrder=1  InputFilterTimeConstant=0.001  UdotUserProvided=0
  Simulink-PS Converter1 : nesl_utility/Simulink-PS Converter  PhysicalDomain=network_engine_domain  SubClassName=ps_input  LeftPortType=input  RightPortType=output  PseudoPeriodic=off  Frequencies=[]  NoiseDistribution=none  NoiseParameters=[]  Unit=1  AffineConversion=off  FilteringAndDerivatives=provide  SimscapeFilterOrder=1  InputFilterTimeConstant=0.001  UdotUserProvided=0
  Simulink-PS Converter3 : nesl_utility/Simulink-PS Converter  PhysicalDomain=network_engine_domain  SubClassName=ps_input  LeftPortType=input  RightPortType=output  PseudoPeriodic=off  Frequencies=[]  NoiseDistribution=none  NoiseParameters=[]  Unit=1  AffineConversion=off  FilteringAndDerivatives=provide  SimscapeFilterOrder=1  InputFilterTimeConstant=0.001  UdotUserProvided=0
  Sum : Sum  Inputs=++|
  Conn1 : PMIOPort  Side=Left
  wires:
  Constant3/1 -> Sum/1
  Constant/1 -> Sum/2
  Constant1/1 -> Product/2
  Constant2/1 -> Product1/2
  Sum/1 -> Simulink-PS Converter1/1
  Product/1 -> Simulink-PS Converter/1
  [N_BDR1] -> Product/1
  [N_BDR1] -> Product1/1
  Product1/1 -> Simulink-PS Converter3/1
  connections:
  Simulink-PS Converter1/RConn1 -- Inhabitant CO2 Gain/RConn2 -- Inhabitant Moisture Gain/RConn2
  Inhabitant Moisture Gain/LConn1 -- Conn1/RConn1 -- Inhabitant CO2 Gain/LConn1
  Simulink-PS Converter3/RConn1 -- Inhabitant CO2 Gain/RConn1
  Simulink-PS Converter/RConn1 -- Inhabitant Moisture Gain/RConn1

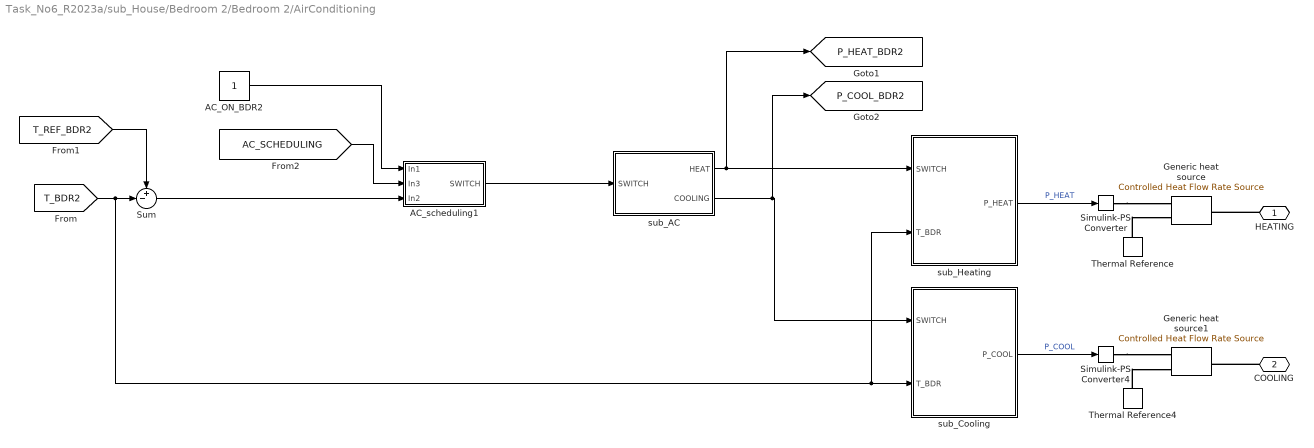
== system Task_No6_R2023a/sub_House/Bedroom 2/Bedroom 2/AirConditioning ==
  AC_ON_BDR2 : Constant
  AC_scheduling1 : Subsystem
  Generic heat source : fl_lib/Thermal/Thermal Sources/Controlled Heat Flow Rate Source
  Generic heat source1 : fl_lib/Thermal/Thermal Sources/Controlled Heat Flow Rate Source
  Simulink-PS Converter : nesl_utility/Simulink-PS Converter  PhysicalDomain=network_engine_domain  SubClassName=ps_input  LeftPortType=input  RightPortType=output  PseudoPeriodic=off  Frequencies=[]  NoiseDistribution=none  NoiseParameters=[]  Unit=1  AffineConversion=off  FilteringAndDerivatives=provide  SimscapeFilterOrder=1  InputFilterTimeConstant=0.001  UdotUserProvided=0
  Simulink-PS Converter4 : nesl_utility/Simulink-PS Converter  PhysicalDomain=network_engine_domain  SubClassName=ps_input  LeftPortType=input  RightPortType=output  PseudoPeriodic=off  Frequencies=[]  NoiseDistribution=none  NoiseParameters=[]  Unit=1  AffineConversion=off  FilteringAndDerivatives=provide  SimscapeFilterOrder=1  InputFilterTimeConstant=0.001  UdotUserProvided=0
  Sum : Sum  Inputs=+-|
  Thermal Reference : fl_lib/Thermal/Thermal Elements/Thermal Reference
  Thermal Reference4 : fl_lib/Thermal/Thermal Elements/Thermal Reference
  sub_AC : Subsystem
  sub_Cooling : Subsystem
  sub_Heating : Subsystem
  HEATING : PMIOPort  Side=Right
  COOLING : PMIOPort  Port=2  Side=Right
  tag scope: P_COOL_BDR2=global, P_HEAT_BDR2=global
  wires:
  sub_AC/2(COOLING) -> [P_COOL_BDR2], sub_Cooling/1(SWITCH)
  sub_AC/1(HEAT) -> [P_HEAT_BDR2], sub_Heating/1(SWITCH)
  [T_BDR2] -> sub_Heating/2(T_BDR), sub_Cooling/2(T_BDR), Sum/2
  sub_Heating/1(P_HEAT) -> Simulink-PS Converter/1  "P_HEAT"
  sub_Cooling/1(P_COOL) -> Simulink-PS Converter4/1  "P_COOL"
  [T_REF_BDR2] -> Sum/1
  Sum/1 -> AC_scheduling1/3(In2)
  AC_scheduling1/1(SWITCH) -> sub_AC/1(SWITCH)
  AC_ON_BDR2/1 -> AC_scheduling1/1(In1)
  [AC_SCHEDULING] -> AC_scheduling1/2(In3)
  connections:
  Thermal Reference4/LConn1 -- Generic heat source1/RConn2
  Thermal Reference/LConn1 -- Generic heat source/RConn2
  Simulink-PS Converter4/RConn1 -- Generic heat source1/RConn1
  Simulink-PS Converter/RConn1 -- Generic heat source/RConn1
  HEATING/RConn1 -- Generic heat source/LConn1
  COOLING/RConn1 -- Generic heat source1/LConn1

== system Task_No6_R2023a/sub_House/Bedroom 2/Bedroom 2/Ceiling & Floor (BDR2<->Above & Below) ==
  Ceiling-InAir : fl_lib/Thermal/Thermal Elements/Thermal Resistance  resistance=1/(U_CEIL*P_AREA_BDR2) K/W  T_specify=off  T_priority=None  T=0 K  T_nominal_specify=off  T_nominal_unit=K  T_nominal_value=1  Q_specify=off  Q_priority=None  Q=0 W  Q_nominal_specify=off  Q_nominal_unit=W  Q_nominal_value=1
  Floor-InAir : fl_lib/Thermal/Thermal Elements/Thermal Resistance  resistance=1/(U_CEIL*P_AREA_BDR2) K/W  T_specify=off  T_priority=None  T=0 K  T_nominal_specify=off  T_nominal_unit=K  T_nominal_value=1  Q_specify=off  Q_priority=None  Q=0 W  Q_nominal_specify=off  Q_nominal_unit=W  Q_nominal_value=1
  Conn1 : PMIOPort  Side=Left
  Conn2 : PMIOPort  Port=2  Side=Right
  connections:
  Conn1/RConn1 -- Ceiling-InAir/LConn1 -- Floor-InAir/LConn1
  Conn2/RConn1 -- Ceiling-InAir/RConn1 -- Floor-InAir/RConn1

== system Task_No6_R2023a/sub_House/Bedroom 2/Bedroom 2/Heat source human ==
  Constant : Constant  Value=P_HUMAN
  Controlled Heat Flow Rate Source : fl_lib/Thermal/Thermal Sources/Controlled Heat Flow Rate Source
  Product : Product
  Simulink-PS Converter : nesl_utility/Simulink-PS Converter  PhysicalDomain=network_engine_domain  SubClassName=ps_input  LeftPortType=input  RightPortType=output  PseudoPeriodic=off  Frequencies=[]  NoiseDistribution=none  NoiseParameters=[]  Unit=1  AffineConversion=off  FilteringAndDerivatives=provide  SimscapeFilterOrder=1  InputFilterTimeConstant=0.001  UdotUserProvided=0
  Thermal Reference : fl_lib/Thermal/Thermal Elements/Thermal Reference
  Conn1 : PMIOPort  Side=Left
  wires:
  [N_BDR2] -> Product/1
  Constant/1 -> Product/2
  Product/1 -> Simulink-PS Converter/1
  connections:
  Thermal Reference/LConn1 -- Controlled Heat Flow Rate Source/RConn2
  Simulink-PS Converter/RConn1 -- Controlled Heat Flow Rate Source/RConn1
  Controlled Heat Flow Rate Source/LConn1 -- Conn1/RConn1

== system Task_No6_R2023a/sub_House/Bedroom 2/Bedroom 2/Inside Enivornment Temperature ==
  T_ENV : Inport
  Constant2 : Constant  Value=Conv_C_to_K
  Controlled Temperature Source : fl_lib/Thermal/Thermal Sources/Controlled Temperature Source
  Simulink-PS Converter1 : nesl_utility/Simulink-PS Converter  PhysicalDomain=network_engine_domain  SubClassName=ps_input  LeftPortType=input  RightPortType=output  PseudoPeriodic=off  Frequencies=[]  NoiseDistribution=none  NoiseParameters=[]  Unit=1  AffineConversion=off  FilteringAndDerivatives=provide  SimscapeFilterOrder=1  InputFilterTimeConstant=0.001  UdotUserProvided=0
  Sum : Sum  Inputs=|++
  Thermal Reference1 : fl_lib/Thermal/Thermal Elements/Thermal Reference
  Conn1 : PMIOPort  Side=Left
  wires:
  T_ENV/1 -> Sum/1
  Constant2/1 -> Sum/2
  Sum/1 -> Simulink-PS Converter1/1
  connections:
  Controlled Temperature Source/LConn1 -- Conn1/RConn1
  Simulink-PS Converter1/RConn1 -- Controlled Temperature Source/RConn1
  Thermal Reference1/LConn1 -- Controlled Temperature Source/RConn2

== system Task_No6_R2023a/sub_House/Bedroom 2/Bedroom 2/Outside Temperature ==
  T_OUT : Inport
  Constant2 : Constant  Value=Conv_C_to_K
  Controlled Temperature Source : fl_lib/Thermal/Thermal Sources/Controlled Temperature Source
  Simulink-PS Converter1 : nesl_utility/Simulink-PS Converter  PhysicalDomain=network_engine_domain  SubClassName=ps_input  LeftPortType=input  RightPortType=output  PseudoPeriodic=off  Frequencies=[]  NoiseDistribution=none  NoiseParameters=[]  Unit=1  AffineConversion=off  FilteringAndDerivatives=provide  SimscapeFilterOrder=1  InputFilterTimeConstant=0.001  UdotUserProvided=0
  Sum : Sum  Inputs=|++
  Thermal Reference1 : fl_lib/Thermal/Thermal Elements/Thermal Reference
  Conn1 : PMIOPort  Side=Left
  wires:
  Sum/1 -> Simulink-PS Converter1/1
  Constant2/1 -> Sum/2
  T_OUT/1 -> Sum/1
  connections:
  Thermal Reference1/LConn1 -- Controlled Temperature Source/RConn2
  Simulink-PS Converter1/RConn1 -- Controlled Temperature Source/RConn1
  Controlled Temperature Source/LConn1 -- Conn1/RConn1

== system Task_No6_R2023a/sub_House/Bedroom 2/Bedroom 2/SOLAR__WALL ==
  Add : Sum
  Constant : Constant  Value=P_AREA_NORTH_WALL_BDR2
  Constant1 : Constant  Value=P_EM_WALL
  Constant2 : Constant  Value=P_AREA_EAST_WALL_BDR2
  Constant3 : Constant  Value=P_EM_WALL
  Controlled Heat Flow Rate Source : fl_lib/Thermal/Thermal Sources/Controlled Heat Flow Rate Source
  Product : Product  Inputs=3
  Product1 : Product  Inputs=3
  Simulink-PS Converter : nesl_utility/Simulink-PS Converter  PhysicalDomain=network_engine_domain  SubClassName=ps_input  LeftPortType=input  RightPortType=output  PseudoPeriodic=off  Frequencies=[]  NoiseDistribution=none  NoiseParameters=[]  Unit=1  AffineConversion=off  FilteringAndDerivatives=provide  SimscapeFilterOrder=1  InputFilterTimeConstant=0.001  UdotUserProvided=0
  Thermal Reference : fl_lib/Thermal/Thermal Elements/Thermal Reference
  Conn1 : PMIOPort  Side=Left
  wires:
  Constant/1 -> Product/2
  Constant1/1 -> Product/1
  [SOL_NORTH] -> Product/3
  Product/1 -> Add/1
  Constant3/1 -> Product1/1
  [SOL_EAST] -> Product1/3
  Constant2/1 -> Product1/2
  Add/1 -> Simulink-PS Converter/1
  Product1/1 -> Add/2
  connections:
  Controlled Heat Flow Rate Source/LConn1 -- Conn1/RConn1
  Simulink-PS Converter/RConn1 -- Controlled Heat Flow Rate Source/RConn1
  Thermal Reference/LConn1 -- Controlled Heat Flow Rate Source/RConn2

== system Task_No6_R2023a/sub_House/Bedroom 2/Bedroom 2/SOLAR__WINDOW ==
  Add : Sum
  Constant : Constant  Value=P_AREA_WIN_BDRS
  Constant1 : Constant  Value=P_EM_GLASS
  Constant2 : Constant  Value=P_AREA_WIN_BDRS
  Constant3 : Constant  Value=P_EM_GLASS
  Controlled Heat Flow Rate Source : fl_lib/Thermal/Thermal Sources/Controlled Heat Flow Rate Source
  Product : Product  Inputs=3
  Product1 : Product  Inputs=3
  Simulink-PS Converter : nesl_utility/Simulink-PS Converter  PhysicalDomain=network_engine_domain  SubClassName=ps_input  LeftPortType=input  RightPortType=output  PseudoPeriodic=off  Frequencies=[]  NoiseDistribution=none  NoiseParameters=[]  Unit=1  AffineConversion=off  FilteringAndDerivatives=provide  SimscapeFilterOrder=1  InputFilterTimeConstant=0.001  UdotUserProvided=0
  Thermal Reference : fl_lib/Thermal/Thermal Elements/Thermal Reference
  Conn1 : PMIOPort  Side=Left
  wires:
  Product/1 -> Add/1
  [SOL_NORTH] -> Product/3
  Constant1/1 -> Product/1
  Constant/1 -> Product/2
  Constant2/1 -> Product1/2
  Constant3/1 -> Product1/1
  [SOL_EAST] -> Product1/3
  Add/1 -> Simulink-PS Converter/1
  Product1/1 -> Add/2
  connections:
  Thermal Reference/LConn1 -- Controlled Heat Flow Rate Source/RConn2
  Simulink-PS Converter/RConn1 -- Controlled Heat Flow Rate Source/RConn1
  Controlled Heat Flow Rate Source/LConn1 -- Conn1/RConn1

== system Task_No6_R2023a/sub_House/Bedroom 2/Bedroom 2/TEMP_01 ==
  Constant2 : Constant  Value=Conv_C_to_K
  PS-Simulink Converter : nesl_utility/PS-Simulink Converter  PhysicalDomain=network_engine_domain  SubClassName=ps_output  LeftPortType=input  RightPortType=output  PseudoPeriodic=off  Frequencies=[]  VectorFormat=inherit  Unit=inherit  AffineConversion=off
  Sum : Sum  Inputs=|+-
  Temperature Sensor : fl_lib/Thermal/Thermal Sensors/Temperature Sensor  temperature_measure=foundation.enum.MeasurementReference.difference
  Thermal Reference2 : fl_lib/Thermal/Thermal Elements/Thermal Reference
  PS : PMIOPort  Side=Left
  Sim : Outport
  wires:
  Constant2/1 -> Sum/2
  PS-Simulink Converter/1 -> Sum/1
  Sum/1 -> Sim/1
  connections:
  PS/RConn1 -- Temperature Sensor/LConn1
  PS-Simulink Converter/LConn1 -- Temperature Sensor/RConn2
  Thermal Reference2/LConn1 -- Temperature Sensor/RConn1

== system Task_No6_R2023a/sub_House/Bedroom 2/Bedroom 2/Wall (BDR2<->Outside) ==
  InAir-Wall : fl_lib/Thermal/Thermal Elements/Thermal Resistance  resistance=1/(U_WALL*P_AREA_OUTER_WALL_BDR2)/2 K/W  T_specify=off  T_priority=None  T=0 K  T_nominal_specify=off  T_nominal_unit=K  T_nominal_value=1  Q_specify=off  Q_priority=None  Q=0 W  Q_nominal_specify=off  Q_nominal_unit=W  Q_nominal_value=1
  Thermal Mass of wall : fl_lib/Thermal/Thermal Elements/Thermal Mass  mass_type=foundation.enum.constant_variable.constant  mass=P_AREA_OUTER_WALL_BDR2*(P_THICK_BRICK*P_DENSITY_BRICK+P_THICK_PUR*P_DENSITY_PUR) kg  sp_heat=P_CP_WALL J/(K*kg)  mass_min=1e-6 kg  num_ports=foundation.enum.numPorts2.one  m_specify=off  m_priority=High  m=1 kg  m_nominal_specify=off  m_nominal_unit=kg  m_nominal_value=1  T_specify=on  T_priority=High  T=T_INIT_BDR degC  T_nominal_specify=off  T_nominal_unit=K  T_nominal_value=1  Q_specify=off  Q_priority=None  Q=0 W  Q_nominal_specify=off  Q_nominal_unit=W  Q_nominal_value=1
  Wall-OutAir : fl_lib/Thermal/Thermal Elements/Thermal Resistance  resistance=1/(U_WALL*P_AREA_OUTER_WALL_BDR2)/2 K/W  T_specify=off  T_priority=None  T=0 K  T_nominal_specify=off  T_nominal_unit=K  T_nominal_value=1  Q_specify=off  Q_priority=None  Q=0 W  Q_nominal_specify=off  Q_nominal_unit=W  Q_nominal_value=1
  Conn1 : PMIOPort  Side=Left
  Conn3 : PMIOPort  Port=2  Side=Right
  Conn2 : PMIOPort  Port=3  Side=Right
  connections:
  Wall-OutAir/RConn1 -- Conn2/RConn1
  Wall-OutAir/LConn1 -- Conn3/RConn1 -- Thermal Mass of wall/LConn1 -- InAir-Wall/RConn1
  Conn1/RConn1 -- InAir-Wall/LConn1
